simulink model "vymennik"  (R2019b)
settings: Solver=VariableStepAuto  StartTime=0.0  StopTime=6  RelTol=1e-3
values from neighbouring files (symbols this model uses):
  B1 = 0.9817    [vymennik1.m]
  B2 = 1.4137    [vymennik1.m]
  cp1 = 4186    [vymennik1.m]
  cp2 = 2420    [vymennik1.m]
  la12 = 1020000    [vymennik1.m]
  la2ok = 21000    [vymennik1.m]
  M1 = 200    [vymennik1.m]
  M2 = 300    [vymennik1.m]
  ro1 = 1000    [vymennik1.m]
  ro2 = 770    [vymennik1.m]
  T1i = 80    [vymennik1.m]
  T2i = 18    [vymennik1.m]
  Tok = 18    [vymennik1.m]
  V1 = 0.0982    [vymennik1.m]
  V2 = 0.0715    [vymennik1.m]
settings Model: Creator=student  LastModifiedBy=student

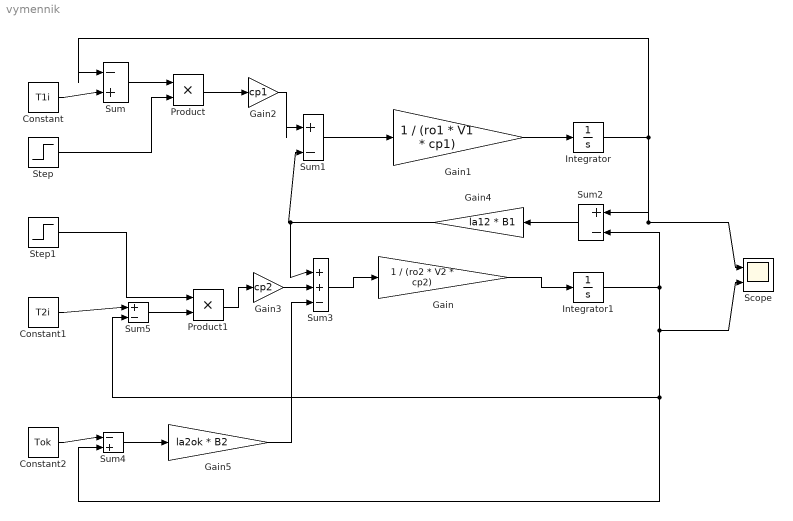
== system vymennik ==
  Constant : Constant  Value=T1i
  Constant1 : Constant  Value=T2i
  Constant2 : Constant  Value=Tok
  Gain : Gain  Gain=1 / (ro2 * V2 * cp2)
  Gain1 : Gain  Gain=1 / (ro1 * V1 * cp1)
  Gain2 : Gain  Gain=cp1
  Gain3 : Gain  Gain=cp2
  Gain4 : Gain  Gain=la12 * B1
  Gain5 : Gain  Gain=la2ok * B2
  Integrator : Integrator  InitialCondition=58.9
  Integrator1 : Integrator  InitialCondition=41.3
  Product : Product
  Product1 : Product
  Scope : Scope  NumInputPorts=2
  Step : Step  Time=3  Before=M1  After=M1/2  SampleTime=0
  Step1 : Step  Time=0.5  Before=M2  After=M2/2  SampleTime=0
  Sum : Sum  Inputs=|-+
  Sum1 : Sum  Inputs=|+-
  Sum2 : Sum  Inputs=|+-
  Sum3 : Sum  Inputs=|++-
  Sum4 : Sum  Inputs=|-+
  Sum5 : Sum  Inputs=|+-
  wires:
  Constant/1 -> Sum/2
  Sum/1 -> Product/1
  Product/1 -> Gain2/1
  Gain2/1 -> Sum1/1
  Sum1/1 -> Gain1/1
  Gain1/1 -> Integrator/1
  Integrator/1 -> Scope/1, Sum2/1, Sum/1
  Step/1 -> Product/2
  Sum2/1 -> Gain4/1
  Gain4/1 -> Sum3/1, Sum1/2
  Sum3/1 -> Gain/1
  Gain/1 -> Integrator1/1
  Integrator1/1 -> Scope/2, Sum4/2, Sum5/2, Sum2/2
  Gain5/1 -> Sum3/3
  Sum4/1 -> Gain5/1
  Constant2/1 -> Sum4/1
  Constant1/1 -> Sum5/1
  Sum5/1 -> Product1/2
  Step1/1 -> Product1/1
  Product1/1 -> Gain3/1
  Gain3/1 -> Sum3/2
